simulink model "sampleModel1"  (R2021a)
settings: Solver=VariableStepAuto  StartTime=0.0  StopTime=50  RelTol=1e-3
undefined symbols (not defined in the file): DiscIntNeverNeededParam, magnitude, Newton, Raphson
libraries: simulink x92, pid_lib x10
(part 4 of 5)

== system sampleModel1/cfblk103/cfblk5/cfblk21/cfblk13 ==
  cfblk1 : Inport
  cfblk10 : Sin  TimeSource=Use external signal  SampleTime=0
  cfblk11 : Constant  Value=[-419511582.432887]  SampleTime=1
  cfblk12 : Constant  Value=[-579938406.585944]  SampleTime=1
  cfblk13 : Constant  Value=[41031774.650466]  SampleTime=1
  cfblk14 : Delay
  cfblk15 : Delay
  cfblk16 : Delay
  cfblk3 : simulink/Discrete/Difference  ICPrevInput=0.0  OutMin=[]  OutMax=[]  OutDataTypeStr=Inherit: Inherit via back propagation  OutDataType=fixdt(1, 16)  OutScaling=2^-10  DoSatur=off
  cfblk4 : UnitDelay  SampleTime=-1  HasFrameUpgradeWarning=on
  cfblk5 : Sum  Inputs=+-
  cfblk6 : MinMax  Function=max  Inputs=3
  cfblk7 : ComplexToRealImag
  cfblk8 : simulink/Math Operations/MinMax Running Resettable  Function=min  vinit=0.0
  cfblk9 : MinMax  Function=max  Inputs=2
  cfblk2 : Outport
  wires:
  cfblk4/1 -> cfblk5/1
  cfblk13/1 -> cfblk2/1
  cfblk6/1 -> cfblk7/1
  cfblk11/1 -> cfblk8/1, cfblk6/3
  cfblk9/1 -> cfblk5/2
  cfblk12/1 -> cfblk4/1
  cfblk7/1 -> cfblk8/2
  cfblk7/2 -> cfblk10/1
  cfblk1/1 -> cfblk9/2
  cfblk5/1 -> cfblk3/1
  cfblk3/1 -> cfblk14/1
  cfblk14/1 -> cfblk9/1
  cfblk8/1 -> cfblk15/1
  cfblk15/1 -> cfblk6/1
  cfblk10/1 -> cfblk16/1
  cfblk16/1 -> cfblk6/2

== system sampleModel1/cfblk103/cfblk5/cfblk9/cfblk13 ==
  cfblk1 : Inport
  cfblk3 : Assignment  DiagnosticForDimensions=Warning  IndexOptions=Index vector (dialog)  Indices=1  OutputSizes=1
  cfblk4 : Constant  Value=[323469888.835887]  SampleTime=1
  cfblk5 : Constant  Value=[-52364273.558147]  SampleTime=1
  cfblk2 : Outport
  cfblk6 : Outport  Port=2
  cfblk7 : Outport  Port=3
  wires:
  cfblk5/1 -> cfblk3/1
  cfblk1/1 -> cfblk7/1
  cfblk4/1 -> cfblk6/1, cfblk3/2
  cfblk3/1 -> cfblk2/1

== system sampleModel1/cfblk104/cfblk18/cfblk9/cfblk8 ==
  cfblk1 : Inport
  cfblk13 : Inport  Port=2
  cfblk14 : Inport  Port=3
  cfblk15 : Inport  Port=4
  cfblk10 : Constant  Value=[468184186.952253]  SampleTime=1
  cfblk11 : Constant  Value=[208357491.204136]  SampleTime=1
  cfblk12 : Constant  Value=[-745066327.969250]  SampleTime=1
  cfblk3 : Product  Inputs=*
  cfblk4 : simulink/Math Operations/MinMax Running Resettable  Function=min  vinit=0.0
  cfblk5 : ComplexToMagnitudeAngle
  cfblk6 : DotProduct  InputSameDT=on  OutDataTypeStr=Inherit: Inherit via internal rule
  cfblk7 : PermuteDimensions
  cfblk8 : Constant  Value=[65566875.393897]  SampleTime=1
  cfblk9 : Constant  Value=[546229624.544757]  SampleTime=1
  cfblk2 : Outport
  cfblk16 : Outport  Port=2
  cfblk17 : Outport  Port=3
  wires:
  cfblk10/1 -> cfblk4/1
  cfblk7/1 -> cfblk17/1
  cfblk15/1 -> cfblk2/1
  cfblk5/1 -> cfblk16/1
  cfblk12/1 -> cfblk4/2
  cfblk9/1 -> cfblk6/1
  cfblk1/1 -> cfblk6/2
  cfblk14/1 -> cfblk7/1
  cfblk13/1 -> cfblk3/1
  cfblk3/1 -> cfblk5/1

== system sampleModel1/cfblk104/cfblk19/cfblk17/cfblk12 ==
  cfblk1 : Inport
  cfblk8 : Inport  Port=2
  cfblk9 : Inport  Port=3
  cfblk10 : Inport  Port=4
  cfblk11 : Inport  Port=5
  cfblk12 : Inport  Port=6
  cfblk3 : Sqrt  Operator=rSqrt  AlgorithmType=Newton-Raphson  SaturateOnIntegerOverflow=on
  cfblk4 : PermuteDimensions
  cfblk5 : Assignment  DiagnosticForDimensions=Warning  IndexOptions=Index vector (dialog)  Indices=1  OutputSizes=1
  cfblk6 : Squeeze
  cfblk7 : Constant  Value=[-465349889.808491]  SampleTime=1
  cfblk2 : Outport
  cfblk13 : Outport  Port=2
  wires:
  cfblk5/1 -> cfblk3/1
  cfblk4/1 -> cfblk5/1
  cfblk10/1 -> cfblk2/1
  cfblk8/1 -> cfblk4/1
  cfblk7/1 -> cfblk5/2
  cfblk3/1 -> cfblk13/1
  cfblk12/1 -> cfblk6/1

== system sampleModel1/cfblk104/cfblk19/cfblk17/cfblk13 ==
  cfblk1 : Inport
  cfblk10 : Constant  Value=[70162531.435561]  SampleTime=1
  cfblk11 : Constant  Value=[340915322.911899]  SampleTime=1
  cfblk12 : Constant  Value=[-734252110.443880]  SampleTime=1
  cfblk13 : Constant  Value=[95285484.546552]  SampleTime=1
  cfblk3 : simulink/Discrete/Transfer Fcn Lead or Lag  PoleZ=0.95  ZeroZ=0.75  ICPrevOutput=0.0  ICPrevInput=0.0  DoSatur=off
      settings: SourceProductBaseCode=SL
  cfblk4 : Delay
  cfblk5 : Sqrt  SaturateOnIntegerOverflow=on
  cfblk6 : Sqrt  SaturateOnIntegerOverflow=on
  cfblk7 : Sin  TimeSource=Use external signal  SampleTime=0
  cfblk8 : Sqrt  Operator=rSqrt  AlgorithmType=Newton-Raphson  SaturateOnIntegerOverflow=on
  cfblk9 : Constant  Value=[329230040.299835]  SampleTime=1
  cfblk2 : Outport
  cfblk14 : Outport  Port=2
  wires:
  cfblk11/1 -> cfblk5/1
  cfblk7/1 -> cfblk6/1
  cfblk4/1 -> cfblk2/1
  cfblk9/1 -> cfblk7/1
  cfblk13/1 -> cfblk8/1
  cfblk1/1 -> cfblk14/1
  cfblk3/1 -> cfblk4/1
  cfblk8/1 -> cfblk3/1

== system sampleModel1/cfblk104/cfblk19/cfblk17/cfblk16 ==
  cfblk1 : Inport
  cfblk7 : Inport  Port=2
  Action Port : ActionPort  ActionPortLabel=if(u1 >= 0)
  cfblk3 : ComplexToMagnitudeAngle
  cfblk4 : Reshape
  cfblk5 : ComplexToRealImag
  cfblk6 : Assignment  DiagnosticForDimensions=Warning  IndexOptions=Index vector (dialog)  Indices=1  OutputSizes=1
  cfblk2 : Outport
  wires:
  cfblk4/1 -> cfblk5/1
  cfblk7/1 -> cfblk3/1
  cfblk5/1 -> cfblk6/1
  cfblk5/2 -> cfblk2/1
  cfblk1/1 -> cfblk4/1
  cfblk3/1 -> cfblk6/2

== system sampleModel1/cfblk104/cfblk19/cfblk17/cfblk17 ==
  cfblk1 : Inport
  cfblk9 : Inport  Port=2
  Action Port : ActionPort  ActionPortLabel=else
  cfblk3 : Sum  Inputs=+-
  cfblk4 : Sin  TimeSource=Use external signal  SampleTime=0
  cfblk5 : Squeeze
  cfblk6 : ComplexToRealImag
  cfblk7 : Constant  Value=[-869127634.488702]  SampleTime=1
  cfblk8 : Constant  Value=[403105618.550086]  SampleTime=1
  cfblk2 : Outport
  wires:
  cfblk6/1 -> cfblk2/1
  cfblk8/1 -> cfblk6/1
  cfblk7/1 -> cfblk3/1
  cfblk4/1 -> cfblk5/1
  cfblk1/1 -> cfblk3/2
  cfblk3/1 -> cfblk4/1

== system sampleModel1/cfblk104/cfblk19/cfblk18/cfblk7 ==
  cfblk1 : Inport
  cfblk9 : Inport  Port=2
  cfblk10 : Inport  Port=3
  cfblk11 : Delay
  cfblk3 : DiscreteFir
  cfblk4 : Reshape
  cfblk5 : Sqrt  Operator=rSqrt  AlgorithmType=Newton-Raphson  SaturateOnIntegerOverflow=on
  cfblk6 : Bias  Bias=[-686765959.780988]
  cfblk7 : Constant  Value=[-130705177.150606]  SampleTime=1
  cfblk8 : Constant  Value=[-280180877.090353]  SampleTime=1
  cfblk2 : Outport
  wires:
  cfblk5/1 -> cfblk4/1
  cfblk8/1 -> cfblk2/1
  cfblk3/1 -> cfblk5/1
  cfblk7/1 -> cfblk6/1
  cfblk4/1 -> cfblk11/1
  cfblk11/1 -> cfblk3/1

== system sampleModel1/cfblk104/cfblk21/cfblk11/cfblk11 ==
  cfblk1 : Inport
  cfblk10 : Inport  Port=2
  cfblk11 : Inport  Port=3
  cfblk3 : DiscreteFir
  cfblk4 : UnitDelay  SampleTime=-1  HasFrameUpgradeWarning=on
  cfblk5 : Abs
  cfblk6 : Sin  TimeSource=Use external signal  SampleTime=0
  cfblk7 : Sqrt  SaturateOnIntegerOverflow=on
  cfblk8 : Constant  Value=[815597882.142010]  SampleTime=1
  cfblk9 : Constant  Value=[-760273017.735555]  SampleTime=1
  cfblk2 : Outport
  wires:
  cfblk8/1 -> cfblk6/1
  cfblk11/1 -> cfblk7/1
  cfblk1/1 -> cfblk5/1
  cfblk5/1 -> cfblk3/1
  cfblk3/1 -> cfblk2/1
  cfblk9/1 -> cfblk4/1

== system sampleModel1/cfblk104/cfblk21/cfblk11/cfblk12 ==
  cfblk1 : Inport
  cfblk10 : Constant  Value=[261499476.768893]  SampleTime=1
  cfblk11 : Constant  Value=[-508647636.126222]  SampleTime=1
  cfblk12 : Constant  Value=[-390080084.785966]  SampleTime=1
  cfblk13 : Constant  Value=[-465541815.265822]  SampleTime=1
  cfblk14 : Constant  Value=[-406876444.934026]  SampleTime=1
  cfblk15 : Constant  Value=[938148942.176117]  SampleTime=1
  cfblk16 : Constant  Value=[435762796.775185]  SampleTime=1
  cfblk3 : simulink/Math Operations/MinMax Running Resettable  Function=min  vinit=0.0
  cfblk4 : Sqrt  SaturateOnIntegerOverflow=on
  cfblk5 : Squeeze
  cfblk6 : simulink/Math Operations/Slider Gain  gain=1  low=0  high=2
  cfblk7 : Sqrt  SaturateOnIntegerOverflow=on
  cfblk8 : Product
  cfblk9 : Product  Inputs=*
  cfblk2 : Outport
  cfblk17 : Outport  Port=2
  wires:
  cfblk15/1 -> cfblk6/1
  cfblk8/1 -> cfblk5/1
  cfblk13/1 -> cfblk3/1
  cfblk5/1 -> cfblk7/1
  cfblk3/1 -> cfblk9/1
  cfblk10/1 -> cfblk2/1
  cfblk11/1 -> cfblk8/1
  cfblk12/1 -> cfblk17/1
  cfblk6/1 -> cfblk4/1
  cfblk14/1 -> cfblk3/2
  cfblk4/1 -> cfblk8/2

== system sampleModel1/cfblk104/cfblk21/cfblk12/cfblk12 ==
  cfblk1 : Inport
  Action Port : ActionPort  ActionPortLabel=if(u1 >= 0)
  cfblk11 : Delay
  cfblk3 : UnitDelay  SampleTime=-1  HasFrameUpgradeWarning=on
  cfblk4 : Rounding
  cfblk5 : MinMax  Inputs=3
  cfblk6 : Constant  Value=[890112149.879811]  SampleTime=1
  cfblk7 : Constant  Value=[-865439630.913288]  SampleTime=1
  cfblk8 : Constant  Value=[151495230.431139]  SampleTime=1
  cfblk9 : Constant  Value=[-417103288.097467]  SampleTime=1
  cfblk2 : Outport
  cfblk10 : Outport  Port=2
  wires:
  cfblk5/1 -> cfblk3/1
  cfblk3/1 -> cfblk4/1
  cfblk7/1 -> cfblk2/1
  cfblk9/1 -> cfblk5/1
  cfblk8/1 -> cfblk10/1
  cfblk1/1 -> cfblk5/3
  cfblk4/1 -> cfblk11/1
  cfblk11/1 -> cfblk5/2

== system sampleModel1/cfblk104/cfblk21/cfblk12/cfblk13 ==
  cfblk1 : Inport
  cfblk6 : Inport  Port=2
  cfblk7 : Inport  Port=3
  Action Port : ActionPort  ActionPortLabel=else
  cfblk3 : Product  Inputs=**
  cfblk4 : Constant  Value=[673329880.555540]  SampleTime=1
  cfblk5 : Constant  Value=[46754945.948073]  SampleTime=1
  cfblk2 : Outport
  cfblk8 : Outport  Port=2
  wires:
  cfblk1/1 -> cfblk8/1
  cfblk6/1 -> cfblk3/1
  cfblk4/1 -> cfblk3/2
  cfblk3/1 -> cfblk2/1

== system sampleModel1/cfblk104/cfblk21/cfblk12/cfblk14 ==
  cfblk1 : Inport
  Action Port : ActionPort  ActionPortLabel=if(u1 >= 0)
  cfblk10 : Product  Inputs=*
  cfblk11 : Constant  Value=[442312619.835425]  SampleTime=1
  cfblk12 : Constant  Value=[189723836.537281]  SampleTime=1
  cfblk13 : Constant  Value=[-102397878.841420]  SampleTime=1
  cfblk16 : Delay
  cfblk3 : Product  Inputs=**
  cfblk4 : PermuteDimensions
  cfblk5 : Bias  Bias=[-155918482.521040]
  cfblk6 : Sqrt  SaturateOnIntegerOverflow=on
  cfblk7 : ComplexToRealImag
  cfblk8 : Sqrt  SaturateOnIntegerOverflow=on
  cfblk9 : Product
  cfblk2 : Outport
  cfblk14 : Outport  Port=2
  cfblk15 : Outport  Port=3
  wires:
  cfblk9/1 -> cfblk5/1
  cfblk11/1 -> cfblk4/1
  cfblk13/1 -> cfblk14/1
  cfblk5/1 -> cfblk7/1
  cfblk3/1 -> cfblk2/1
  cfblk12/1 -> cfblk15/1
  cfblk7/1 -> cfblk8/1
  cfblk7/2 -> cfblk10/1
  cfblk4/1 -> cfblk6/1
  cfblk8/1 -> cfblk3/1
  cfblk6/1 -> cfblk3/2
  cfblk1/1 -> cfblk9/2
  cfblk10/1 -> cfblk16/1
  cfblk16/1 -> cfblk9/1

== system sampleModel1/cfblk104/cfblk21/cfblk12/cfblk15 ==
  cfblk1 : Inport
  cfblk13 : Inport  Port=2
  cfblk14 : Inport  Port=3
  cfblk15 : Inport  Port=4
  Action Port : ActionPort  ActionPortLabel=else
  cfblk10 : Constant  Value=[-421838795.697533]  SampleTime=1
  cfblk11 : Constant  Value=[-352587754.567201]  SampleTime=1
  cfblk12 : Constant  Value=[-400732601.566113]  SampleTime=1
  cfblk3 : Squeeze
  cfblk4 : ComplexToRealImag
  cfblk5 : Constant  Value=[-948653583.363454]  SampleTime=1
  cfblk6 : Constant  Value=[-714128839.414161]  SampleTime=1
  cfblk7 : Constant  Value=[251689562.661298]  SampleTime=1
  cfblk8 : Constant  Value=[-55335469.502435]  SampleTime=1
  cfblk9 : Constant  Value=[-770422061.669483]  SampleTime=1
  cfblk2 : Outport
  cfblk16 : Outport  Port=2
  wires:
  cfblk10/1 -> cfblk4/1
  cfblk13/1 -> cfblk16/1
  cfblk4/1 -> cfblk3/1
  cfblk4/2 -> cfblk2/1

== system sampleModel1/cfblk105/cfblk6/cfblk10/cfblk10 ==
  cfblk1 : Inport
  cfblk9 : Inport  Port=2
  cfblk11 : Delay
  cfblk12 : Delay
  cfblk3 : ComplexToMagnitudeAngle
  cfblk4 : Sum  Inputs=-+
  cfblk5 : Reshape
  cfblk6 : Signum
  cfblk7 : Sum  Inputs=--
  cfblk8 : Abs
  cfblk2 : Outport
  cfblk10 : Outport  Port=2
  wires:
  cfblk4/1 -> cfblk6/1
  cfblk1/1 -> cfblk10/1
  cfblk8/1 -> cfblk4/2
  cfblk6/1 -> cfblk5/1
  cfblk3/1 -> cfblk8/1
  cfblk9/1 -> cfblk2/1, cfblk7/2
  cfblk3/2 -> cfblk7/1
  cfblk5/1 -> cfblk11/1
  cfblk11/1 -> cfblk4/1
  cfblk7/1 -> cfblk12/1
  cfblk12/1 -> cfblk3/1

== system sampleModel1/cfblk105/cfblk6/cfblk10/cfblk14 ==
  cfblk1 : Inport
  cfblk12 : Inport  Port=2
  cfblk13 : Inport  Port=3
  cfblk14 : Inport  Port=4
  Action Port : ActionPort  ActionPortLabel=if(u1 >= 0)
  cfblk10 : Constant  Value=[909353169.805887]  SampleTime=1
  cfblk11 : Constant  Value=[-627523588.483763]  SampleTime=1
  cfblk3 : simulink/Discrete/Transfer Fcn First Order  PoleZ=0.95  ICPrevOutput=0.0  DoSatur=off
  cfblk4 : Delay
  cfblk5 : Polyval  Coefs=[ +2.081618890e-019, -1.441693666e-014, +4.719686976e-010, -8.536869453e-006, +1.621573104e-001, -8.087801117e+001 ]
  cfblk6 : Product  Inputs=**
  cfblk7 : Product
  cfblk8 : UnaryMinus
  cfblk9 : Constant  Value=[996327052.148197]  SampleTime=1
  cfblk2 : Outport
  cfblk15 : Outport  Port=2
  cfblk16 : Outport  Port=3
  wires:
  cfblk1/1 -> cfblk3/1
  cfblk3/1 -> cfblk8/1
  cfblk9/1 -> cfblk16/1
  cfblk12/1 -> cfblk5/1
  cfblk7/1 -> cfblk15/1
  cfblk11/1 -> cfblk6/1
  cfblk10/1 -> cfblk7/1
  cfblk14/1 -> cfblk4/1
  cfblk8/1 -> cfblk2/1
  cfblk5/1 -> cfblk7/2
  cfblk13/1 -> cfblk6/2

== system sampleModel1/cfblk105/cfblk6/cfblk10/cfblk15 ==
  cfblk1 : Inport
  cfblk9 : Inport  Port=2
  Action Port : ActionPort  ActionPortLabel=else
  cfblk3 : simulink/Discrete/Transfer Fcn Real Zero  ZeroZ=0.75  ICPrevInput=0.0  DoSatur=off
      settings: SourceProductBaseCode=SL
  cfblk4 : Reshape
  cfblk5 : Reshape
  cfblk6 : Constant  Value=[-408517177.426848]  SampleTime=1
  cfblk7 : Constant  Value=[-412588011.215259]  SampleTime=1
  cfblk8 : Constant  Value=[-308205238.166373]  SampleTime=1
  cfblk2 : Outport
  cfblk10 : Outport  Port=2
  cfblk11 : Outport  Port=3
  wires:
  cfblk3/1 -> cfblk2/1
  cfblk7/1 -> cfblk5/1
  cfblk6/1 -> cfblk3/1
  cfblk8/1 -> cfblk11/1
  cfblk1/1 -> cfblk4/1
  cfblk5/1 -> cfblk10/1

== system sampleModel1/cfblk111/cfblk11/cfblk11/cfblk9 ==
  cfblk1 : Inport
  cfblk9 : Inport  Port=2
  cfblk10 : Delay
  cfblk11 : Delay
  cfblk3 : DotProduct  InputSameDT=on  OutDataTypeStr=Inherit: Inherit via internal rule
  cfblk4 : Sum  Inputs=+
  cfblk5 : Trigonometry
  cfblk6 : Sum
  cfblk7 : Sqrt  Operator=rSqrt  AlgorithmType=Newton-Raphson  SaturateOnIntegerOverflow=on
  cfblk8 : Constant  Value=[680678842.980550]  SampleTime=1
  cfblk2 : Outport
  wires:
  cfblk9/1 -> cfblk3/1
  cfblk3/1 -> cfblk7/1
  cfblk4/1 -> cfblk2/1
  cfblk8/1 -> cfblk4/1
  cfblk1/1 -> cfblk6/2
  cfblk6/1 -> cfblk5/1
  cfblk5/1 -> cfblk10/1
  cfblk10/1 -> cfblk6/1
  cfblk7/1 -> cfblk11/1
  cfblk11/1 -> cfblk3/2

== system sampleModel1/cfblk111/cfblk11/cfblk12/cfblk12 ==
  cfblk1 : Inport
  cfblk11 : Inport  Port=2
  Action Port : ActionPort  ActionPortLabel=if(u1 >= 0)
  cfblk10 : Constant  Value=[246879671.288015]  SampleTime=1
  cfblk3 : Polyval  Coefs=[ +2.081618890e-019, -1.441693666e-014, +4.719686976e-010, -8.536869453e-006, +1.621573104e-001, -8.087801117e+001 ]
  cfblk4 : Sqrt  Operator=rSqrt  AlgorithmType=Newton-Raphson  SaturateOnIntegerOverflow=on
  cfblk5 : Sum  Inputs=--
  cfblk6 : Product
  cfblk7 : Reshape
  cfblk8 : Polyval  Coefs=[ +2.081618890e-019, -1.441693666e-014, +4.719686976e-010, -8.536869453e-006, +1.621573104e-001, -8.087801117e+001 ]
  cfblk9 : Constant  Value=[382037661.110754]  SampleTime=1
  cfblk2 : Outport
  cfblk12 : Outport  Port=2
  cfblk13 : Outport  Port=3
  cfblk14 : Outport  Port=4
  cfblk15 : Outport  Port=5
  wires:
  cfblk7/1 -> cfblk3/1
  cfblk6/1 -> cfblk14/1
  cfblk3/1 -> cfblk12/1
  cfblk11/1 -> cfblk8/1, cfblk5/2
  cfblk8/1 -> cfblk4/1
  cfblk4/1 -> cfblk2/1, cfblk5/1
  cfblk10/1 -> cfblk13/1
  cfblk1/1 -> cfblk6/1, cfblk6/2
  cfblk5/1 -> cfblk15/1
  cfblk9/1 -> cfblk7/1

== system sampleModel1/cfblk111/cfblk11/cfblk12/cfblk13 ==
  cfblk1 : Inport
  cfblk13 : Inport  Port=2
  cfblk14 : Inport  Port=3
  Action Port : ActionPort  ActionPortLabel=else
  cfblk10 : Constant  Value=[360855934.077704]  SampleTime=1
  cfblk11 : Constant  Value=[-216363340.487875]  SampleTime=1
  cfblk12 : Constant  Value=[449040613.713941]  SampleTime=1
  cfblk16 : Delay
  cfblk3 : Product  Inputs=*
  cfblk4 : Reshape
  cfblk5 : Squeeze
  cfblk6 : Sqrt  SaturateOnIntegerOverflow=on
  cfblk7 : Assignment  DiagnosticForDimensions=Warning  IndexOptions=Index vector (dialog)  Indices=1  OutputSizes=1
  cfblk8 : Constant  Value=[339926434.778656]  SampleTime=1
  cfblk9 : Constant  Value=[338991206.712136]  SampleTime=1
  cfblk2 : Outport
  cfblk15 : Outport  Port=2
  wires:
  cfblk8/1 -> cfblk15/1
  cfblk10/1 -> cfblk3/1
  cfblk6/1 -> cfblk2/1
  cfblk5/1 -> cfblk7/1
  cfblk11/1 -> cfblk6/1
  cfblk7/1 -> cfblk4/1
  cfblk1/1 -> cfblk5/1
  cfblk4/1 -> cfblk16/1
  cfblk16/1 -> cfblk7/2

== system sampleModel1/cfblk111/cfblk11/cfblk12/cfblk14 ==
  cfblk1 : Inport
  cfblk9 : Inport  Port=2
  Action Port : ActionPort  ActionPortLabel=if(u1 >= 0)
  cfblk3 : Bias  Bias=[-707875719.304627]
  cfblk4 : Assignment  DiagnosticForDimensions=Warning  IndexOptions=Index vector (dialog)  Indices=1  OutputSizes=1
  cfblk5 : Rounding
  cfblk6 : Trigonometry
  cfblk7 : Constant  Value=[387925857.128569]  SampleTime=1
  cfblk8 : Constant  Value=[-912553202.260724]  SampleTime=1
  cfblk2 : Outport
  cfblk10 : Outport  Port=2
  cfblk11 : Outport  Port=3
  wires:
  cfblk5/1 -> cfblk11/1
  cfblk1/1 -> cfblk4/1
  cfblk7/1 -> cfblk3/1
  cfblk4/1 -> cfblk6/1
  cfblk3/1 -> cfblk5/1
  cfblk6/1 -> cfblk10/1
  cfblk9/1 -> cfblk2/1
  cfblk8/1 -> cfblk4/2

== system sampleModel1/cfblk111/cfblk11/cfblk12/cfblk15 ==
  cfblk1 : Inport
  cfblk8 : Inport  Port=2
  cfblk9 : Inport  Port=3
  cfblk10 : Inport  Port=4
  Action Port : ActionPort  ActionPortLabel=else
  cfblk3 : MinMax
  cfblk4 : Signum
  cfblk5 : Rounding
  cfblk6 : Signum
  cfblk7 : Constant  Value=[527812762.659028]  SampleTime=1
  cfblk2 : Outport
  cfblk11 : Outport  Port=2
  wires:
  cfblk10/1 -> cfblk6/1
  cfblk3/1 -> cfblk11/1
  cfblk8/1 -> cfblk4/1
  cfblk6/1 -> cfblk3/1
  cfblk7/1 -> cfblk5/1
  cfblk4/1 -> cfblk2/1

== system sampleModel1/cfblk111/cfblk11/cfblk6/cfblk8 ==
  cfblk1 : Inport
  cfblk8 : Inport  Port=2
  Action Port : ActionPort  ActionPortLabel=if(u1 >= 0)
  cfblk3 : MinMax  Function=max  Inputs=3
  cfblk4 : simulink/Math Operations/Slider Gain  gain=1  low=0  high=2
  cfblk5 : Gain  Gain=[-580713354.556811]
  cfblk6 : Constant  Value=[-39287024.177822]  SampleTime=1
  cfblk7 : Constant  Value=[-735260719.939917]  SampleTime=1
  cfblk2 : Outport
  wires:
  cfblk6/1 -> cfblk2/1
  cfblk7/1 -> cfblk4/1
  cfblk8/1 -> cfblk5/1
  cfblk5/1 -> cfblk3/1
  cfblk4/1 -> cfblk3/2
  cfblk1/1 -> cfblk3/3

== system sampleModel1/cfblk111/cfblk11/cfblk6/cfblk9 ==
  cfblk1 : Inport
  cfblk9 : Inport  Port=2
  cfblk10 : Inport  Port=3
  cfblk11 : Inport  Port=4
  cfblk12 : Inport  Port=5
  Action Port : ActionPort  ActionPortLabel=else
  cfblk15 : Delay
  cfblk3 : PermuteDimensions
  cfblk4 : Bias  Bias=[939018646.363341]
  cfblk5 : Product  Inputs=*
  cfblk6 : Constant  Value=[-115719020.520580]  SampleTime=1
  cfblk7 : Constant  Value=[-778059505.794407]  SampleTime=1
  cfblk8 : Constant  Value=[-674071793.832320]  SampleTime=1
  cfblk2 : Outport
  cfblk13 : Outport  Port=2
  cfblk14 : Outport  Port=3
  wires:
  cfblk3/1 -> cfblk4/1
  cfblk8/1 -> cfblk14/1
  cfblk4/1 -> cfblk5/1
  cfblk7/1 -> cfblk2/1
  cfblk9/1 -> cfblk13/1
  cfblk5/1 -> cfblk15/1
  cfblk15/1 -> cfblk3/1

== system sampleModel1/cfblk111/cfblk11/cfblk7/cfblk12 ==
  cfblk1 : Inport
  cfblk13 : Inport  Port=2
  cfblk14 : Inport  Port=3
  cfblk15 : Inport  Port=4
  cfblk16 : Inport  Port=5
  cfblk10 : Reshape
  cfblk11 : ComplexToRealImag
  cfblk12 : Constant  Value=[-423829694.747288]  SampleTime=1
  cfblk3 : pid_lib/PID Controller  Controller=PID  Form=Parallel  TimeDomain=Discrete-time  UseExternalTs=off  SampleTime=-1  IntegratorMethod=Forward Euler  FilterMethod=Forward Euler  ControllerParametersSource=internal  P=1  I=1  D=0  UseFilter=on  N=100  TunerSelectOption=Transfer Function Based (PID Tuner App)  InitialConditionSource=internal  InitialConditionForIntegrator=0  InitialConditionForFilter=0  DifferentiatorICPrevScaledInput=0  ExternalReset=none  TrackingMode=off  Kt=1  LimitOutput=off  SatLimitsSource=internal  UpperSaturationLimit=inf  LowerSaturationLimit=-inf  LinearizeAsGain=off  AntiWindupMode=none  Kb=1  POutMin=[]  POutMax=[]  IOutMin=[]  IOutMax=[]  DOutMin=[]  DOutMax=[]  NOutMin=[]  NOutMax=[]  SumOutMin=[]  SumOutMax=[]  SaturationOutMin=[]  SaturationOutMax=[]  PParamMin=[]  PParamMax=[]  IParamMin=[]  IParamMax=[]  DParamMin=[]  DParamMax=[]  NParamMin=[]  NParamMax=[]  KbParamMin=[]  KbParamMax=[]  KtParamMin=[]  KtParamMax=[]  KbOutMin=[]  KbOutMax=[]  KtOutMin=[]  KtOutMax=[]  IntegratorOutMin=[]  IntegratorOutMax=[]  FilterOutMin=[]  FilterOutMax=[]  SumI1OutMin=[]  SumI1OutMax=[]  SumI2OutMin=[]  SumI2OutMax=[]  SumI3OutMin=[]  SumI3OutMax=[]  SumI4OutMin=[]  SumI4OutMax=[]  SumDOutMin=[]  SumDOutMax=[]  DifferentiatorOutMin=[]  DifferentiatorOutMax=[]  FilterDiffOutCoefMin=[]  FilterDiffOutCoefMax=[]  ReciprocalOutMin=[]  ReciprocalOutMax=[]  SumDenOutMin=[]  SumDenOutMax=[]  SumNumOutMin=[]  SumNumOutMax=[]  DivideOutMin=[]  DivideOutMax=[]  UdiffTsProdOutMin=[]  UdiffTsProdOutMax=[]  NTsProdOutMin=[]  NTsProdOutMax=[]  UintegralTsProdOutMin=[]  UintegralTsProdOutMax=[]  UngainTsProdOutMin=[]  UngainTsProdOutMax=[]  IntegratorContinuousStateAttributes=''  IntegratorStateMustResolveToSignalObject=off  IntegratorRTWStateStorageClass=Auto  FilterContinuousStateAttributes=''  FilterStateMustResolveToSignalObject=off  FilterRTWStateStorageClass=Auto  ParallelPVariant=InternalParameters  IdealPVariant=Disabled  IVariant=InternalParameters  DVariant=InternalParameters  IntegratorVariant=Discrete  SatVariant=Disabled  AWVariant=Passthrough  PCopyVariant=Disabled  TRVariant=Disabled  FdbkBlocksVariant=Forward  IdealPFdbkVariant=Disabled  SatFdbkVariant=Disabled  DerivativeFilterVariant=ForwardEulerFilter  NVariant=InternalParameters  NCopyVariant=Disabled  FilterICVariant=InternalICsFilter  IntegratorICVariant=InternalICs  ExternalResetVariant=Disabled  TRSumVariant=Passthrough  SumFdbkVariant=Disabled  SumVariant=Sum_PID  TsampFilterVariant=InternalTs  TsampNgainVariant=Passthrough  TsampIntegralVariant=Passthrough  ExternalSaturationOutDataTypeStr=Inherit: Same as second input
  cfblk4 : DiscreteFir
  cfblk5 : Math  Operator=hypot  SaturateOnIntegerOverflow=on
  cfblk6 : Assignment  DiagnosticForDimensions=Warning  IndexOptions=Index vector (dialog)  Indices=1  OutputSizes=1
  cfblk7 : PermuteDimensions
  cfblk8 : PermuteDimensions
  cfblk9 : Sum  Inputs=-+
  cfblk2 : Outport
  wires:
  cfblk4/1 -> cfblk3/1
  cfblk8/1 -> cfblk7/1
  cfblk11/1 -> cfblk10/1
  cfblk10/1 -> cfblk9/1
  cfblk1/1 -> cfblk2/1
  cfblk9/1 -> cfblk4/1
  cfblk5/1 -> cfblk9/2
  cfblk14/1 -> cfblk6/1
  cfblk11/2 -> cfblk6/2
  cfblk7/1 -> cfblk5/1
  cfblk16/1 -> cfblk11/1
  cfblk13/1 -> cfblk5/2
  cfblk15/1 -> cfblk8/1

== system sampleModel1/cfblk111/cfblk11/cfblk7/cfblk13 ==
  cfblk1 : Inport
  cfblk12 : Inport  Port=2
  cfblk13 : Inport  Port=3
  cfblk10 : Constant  Value=[949658750.222794]  SampleTime=1
  cfblk11 : Constant  Value=[-319797678.233112]  SampleTime=1
  cfblk3 : simulink/Discrete/Transfer Fcn Real Zero  ZeroZ=0.75  ICPrevInput=0.0  DoSatur=off
      settings: SourceProductBaseCode=SL
  cfblk4 : Sqrt  Operator=rSqrt  AlgorithmType=Newton-Raphson  SaturateOnIntegerOverflow=on
  cfblk5 : Abs
  cfblk6 : Math  Operator=log  SaturateOnIntegerOverflow=on
  cfblk7 : Product  Inputs=*
  cfblk8 : Reshape
  cfblk9 : PermuteDimensions
  cfblk2 : Outport
  wires:
  cfblk1/1 -> cfblk4/1
  cfblk12/1 -> cfblk6/1
  cfblk13/1 -> cfblk8/1
  cfblk7/1 -> cfblk3/1
  cfblk5/1 -> cfblk2/1
  cfblk8/1 -> cfblk7/1
  cfblk3/1 -> cfblk5/1
  cfblk11/1 -> cfblk9/1

== system sampleModel1/cfblk112/cfblk11/cfblk13/cfblk15 ==
  cfblk1 : Inport
  cfblk11 : Inport  Port=2
  cfblk12 : Inport  Port=3
  cfblk13 : Inport  Port=4
  cfblk14 : Inport  Port=5
  Action Port : ActionPort  ActionPortLabel=if(u1 >= 0)
  cfblk10 : Constant  Value=[-122266068.845746]  SampleTime=1
  cfblk3 : pid_lib/PID Controller (2DOF)  Controller=PID  Form=Parallel  TimeDomain=Discrete-time  UseExternalTs=off  SampleTime=-1  IntegratorMethod=Forward Euler  FilterMethod=Forward Euler  ControllerParametersSource=internal  P=1  I=1  D=0  UseFilter=on  N=100  b=1  c=1  TunerSelectOption=Transfer Function Based (PID Tuner App)  InitialConditionSource=internal  InitialConditionForIntegrator=0  InitialConditionForFilter=0  DifferentiatorICPrevScaledInput=0  ExternalReset=none  TrackingMode=off  Kt=1  LimitOutput=off  SatLimitsSource=internal  UpperSaturationLimit=inf  LowerSaturationLimit=-inf  LinearizeAsGain=off  AntiWindupMode=none  Kb=1  POutMin=[]  POutMax=[]  IOutMin=[]  IOutMax=[]  DOutMin=[]  DOutMax=[]  NOutMin=[]  NOutMax=[]  bOutMin=[]  bOutMax=[]  cOutMin=[]  cOutMax=[]  SumOutMin=[]  SumOutMax=[]  SaturationOutMin=[]  SaturationOutMax=[]  PParamMin=[]  PParamMax=[]  IParamMin=[]  IParamMax=[]  DParamMin=[]  DParamMax=[]  NParamMin=[]  NParamMax=[]  bParamMin=[]  bParamMax=[]  cParamMin=[]  cParamMax=[]  KbParamMin=[]  KbParamMax=[]  KtParamMin=[]  KtParamMax=[]  KbOutMin=[]  KbOutMax=[]  KtOutMin=[]  KtOutMax=[]  IntegratorOutMin=[]  IntegratorOutMax=[]  FilterOutMin=[]  FilterOutMax=[]  SumI1OutMin=[]  SumI1OutMax=[]  SumI2OutMin=[]  SumI2OutMax=[]  SumI3OutMin=[]  SumI3OutMax=[]  SumI4OutMin=[]  SumI4OutMax=[]  SumDOutMin=[]  SumDOutMax=[]  Sum1OutMin=[]  Sum1OutMax=[]  Sum2OutMin=[]  Sum2OutMax=[]  Sum3OutMin=[]  Sum3OutMax=[]  DifferentiatorOutMin=[]  DifferentiatorOutMax=[]  FilterDiffOutCoefMin=[]  FilterDiffOutCoefMax=[]  ReciprocalOutMin=[]  ReciprocalOutMax=[]  SumDenOutMin=[]  SumDenOutMax=[]  SumNumOutMin=[]  SumNumOutMax=[]  DivideOutMin=[]  DivideOutMax=[]  UdiffTsProdOutMin=[]  UdiffTsProdOutMax=[]  NTsProdOutMin=[]  NTsProdOutMax=[]  UintegralTsProdOutMin=[]  UintegralTsProdOutMax=[]  UngainTsProdOutMin=[]  UngainTsProdOutMax=[]  IntegratorContinuousStateAttributes=''  IntegratorStateMustResolveToSignalObject=off  IntegratorRTWStateStorageClass=Auto  FilterContinuousStateAttributes=''  FilterStateMustResolveToSignalObject=off  FilterRTWStateStorageClass=Auto  ParallelPVariant=InternalParameters  IdealPVariant=Disabled  IVariant=InternalParameters  DVariant=InternalParameters  bVariant=InternalParameters  cVariant=InternalParameters  IntegratorVariant=Discrete  SatVariant=Disabled  AWVariant=Passthrough  PCopyVariant=Disabled  TRVariant=Disabled  FdbkBlocksVariant=Forward  IdealPFdbkVariant=Disabled  SatFdbkVariant=Disabled  DerivativeFilterVariant=ForwardEulerFilter  NVariant=InternalParameters  NCopyVariant=Disabled  FilterICVariant=InternalICsFilter  IntegratorICVariant=InternalICs  ExternalResetVariant=Disabled  TRSumVariant=Passthrough  SumFdbkVariant=Disabled  SumVariant=Sum_PID  TsampFilterVariant=InternalTs  TsampNgainVariant=Passthrough  TsampIntegralVariant=Passthrough  ExternalSaturationOutDataTypeStr=Inherit: Same as second input
      settings: SourceProductBaseCode=SL
  cfblk4 : Delay  DelayLengthSource=Input port
      settings: InputPortMap=u0,p1
  cfblk5 : Squeeze
  cfblk6 : Abs
  cfblk7 : ComplexToMagnitudeAngle
  cfblk8 : Polyval  Coefs=[ +2.081618890e-019, -1.441693666e-014, +4.719686976e-010, -8.536869453e-006, +1.621573104e-001, -8.087801117e+001 ]
  cfblk9 : Constant  Value=[161236866.906013]  SampleTime=1
  cfblk2 : Outport
  cfblk15 : Outport  Port=2
  wires:
  cfblk14/1 -> cfblk3/1
  cfblk12/1 -> cfblk4/1
  cfblk6/1 -> cfblk2/1
  cfblk5/1 -> cfblk3/2
  cfblk11/1 -> cfblk15/1
  cfblk8/1 -> cfblk4/2
  cfblk13/1 -> cfblk6/1
  cfblk9/1 -> cfblk5/1
  cfblk4/1 -> cfblk7/1
  cfblk1/1 -> cfblk8/1

== system sampleModel1/cfblk112/cfblk11/cfblk13/cfblk16 ==
  cfblk1 : Inport
  cfblk8 : Inport  Port=2
  Action Port : ActionPort  ActionPortLabel=else
  cfblk3 : Delay
  cfblk4 : PermuteDimensions
  cfblk5 : Squeeze
  cfblk6 : Constant  Value=[743771143.403290]  SampleTime=1
  cfblk7 : Constant  Value=[-527989586.242749]  SampleTime=1
  cfblk2 : Outport
  cfblk9 : Outport  Port=2
  wires:
  cfblk6/1 -> cfblk4/1
  cfblk1/1 -> cfblk2/1
  cfblk8/1 -> cfblk9/1
  cfblk7/1 -> cfblk3/1
  cfblk4/1 -> cfblk5/1

== system sampleModel1/cfblk112/cfblk11/cfblk14/cfblk14 ==
  cfblk1 : Inport
  Action Port : ActionPort  ActionPortLabel=if(u1 >= 0)
  cfblk3 : Squeeze
  cfblk4 : Bias  Bias=[-497638596.073755]
  cfblk5 : Constant  Value=[875215033.780837]  SampleTime=1
  cfblk6 : Constant  Value=[505821738.043894]  SampleTime=1
  cfblk7 : Constant  Value=[-903146563.627624]  SampleTime=1
  cfblk8 : Constant  Value=[450978110.814705]  SampleTime=1
  cfblk9 : Constant  Value=[265114518.304006]  SampleTime=1
  cfblk2 : Outport
  wires:
  cfblk8/1 -> cfblk4/1
  cfblk4/1 -> cfblk2/1
  cfblk1/1 -> cfblk3/1

== system sampleModel1/cfblk112/cfblk11/cfblk14/cfblk15 ==
  cfblk1 : Inport
  Action Port : ActionPort  ActionPortLabel=else
  cfblk10 : Constant  Value=[818202627.503632]  SampleTime=1
  cfblk11 : Constant  Value=[497271600.581116]  SampleTime=1
  cfblk3 : DiscreteIntegrator  SampleTime=-1  ICPrevOutput=DiscIntNeverNeededParam  ICPrevScaledInput=DiscIntNeverNeededParam
  cfblk4 : Sum  Inputs=|++
  cfblk5 : simulink/Math Operations/Slider Gain  gain=1  low=0  high=2
  cfblk6 : Bias  Bias=[-9164173.785582]
  cfblk7 : Polyval  Coefs=[ +2.081618890e-019, -1.441693666e-014, +4.719686976e-010, -8.536869453e-006, +1.621573104e-001, -8.087801117e+001 ]
  cfblk8 : Signum
  cfblk9 : Constant  Value=[-373032670.560984]  SampleTime=1
  cfblk2 : Outport
  wires:
  cfblk4/1 -> cfblk2/1
  cfblk9/1 -> cfblk6/1
  cfblk1/1 -> cfblk8/1
  cfblk7/1 -> cfblk3/1
  cfblk3/1 -> cfblk4/1
  cfblk6/1 -> cfblk7/1
  cfblk10/1 -> cfblk5/1
  cfblk8/1 -> cfblk4/2

== system sampleModel1/cfblk115/cfblk14/cfblk14/cfblk10 ==
  cfblk1 : Inport
  cfblk12 : Inport  Port=2
  cfblk13 : Inport  Port=3
  cfblk10 : Constant  Value=[352581508.259771]  SampleTime=1
  cfblk11 : Constant  Value=[407353705.186988]  SampleTime=1
  cfblk3 : DiscreteZeroPole  Poles=[0 0.5]  Gain=1  SampleTime=-1
  cfblk4 : Trigonometry
  cfblk5 : Product
  cfblk6 : Constant  Value=[346727033.922065]  SampleTime=1
  cfblk7 : Constant  Value=[-837077149.604303]  SampleTime=1
  cfblk8 : Constant  Value=[-431621581.043910]  SampleTime=1
  cfblk9 : Constant  Value=[-541796869.991993]  SampleTime=1
  cfblk2 : Outport
  cfblk14 : Outport  Port=2
  wires:
  cfblk1/1 -> cfblk5/1
  cfblk13/1 -> cfblk4/1
  cfblk8/1 -> cfblk2/1
  cfblk4/1 -> cfblk14/1
  cfblk3/1 -> cfblk5/2
  cfblk7/1 -> cfblk3/1

== system sampleModel1/cfblk115/cfblk14/cfblk14/cfblk7 ==
  cfblk1 : Inport
  cfblk9 : Inport  Port=2
  cfblk10 : Inport  Port=3
  cfblk11 : Inport  Port=4
  cfblk3 : Delay
  cfblk4 : DiscreteStateSpace  SampleTime=-1
  cfblk5 : Sqrt  SaturateOnIntegerOverflow=on
  cfblk6 : Math  Operator=10^u  SaturateOnIntegerOverflow=on
  cfblk7 : Abs
  cfblk8 : Constant  Value=[421829800.069585]  SampleTime=1
  cfblk2 : Outport
  wires:
  cfblk9/1 -> cfblk7/1
  cfblk11/1 -> cfblk2/1
  cfblk1/1 -> cfblk5/1
  cfblk5/1 -> cfblk6/1
  cfblk4/1 -> cfblk3/1
  cfblk8/1 -> cfblk4/1

== system sampleModel1/cfblk115/cfblk14/cfblk14/cfblk8 ==
  cfblk1 : Inport
  cfblk3 : Sum  Inputs=+-
  cfblk4 : Rounding
  cfblk5 : Product
  cfblk6 : Constant  Value=[931029808.892571]  SampleTime=1
  cfblk7 : Constant  Value=[-506641103.816327]  SampleTime=1
  cfblk8 : Constant  Value=[518610889.480997]  SampleTime=1
  cfblk2 : Outport
  cfblk9 : Outport  Port=2
  wires:
  cfblk8/1 -> cfblk9/1
  cfblk1/1 -> cfblk4/1
  cfblk3/1 -> cfblk2/1
  cfblk6/1 -> cfblk5/1
  cfblk4/1 -> cfblk5/2
  cfblk5/1 -> cfblk3/1
  cfblk7/1 -> cfblk3/2

== system sampleModel1/cfblk115/cfblk14/cfblk14/cfblk9 ==
  cfblk1 : Inport
  cfblk10 : Inport  Port=2
  cfblk11 : Inport  Port=3
  cfblk12 : Inport  Port=4
  cfblk13 : Inport  Port=5
  cfblk3 : Gain  Gain=[407057180.554464]
  cfblk4 : PermuteDimensions
  cfblk5 : Product
  cfblk6 : Product  Inputs=*
  cfblk7 : Math  Operator=hermitian  SaturateOnIntegerOverflow=on
  cfblk8 : Constant  Value=[188349514.589146]  SampleTime=1
  cfblk9 : Constant  Value=[477462067.720349]  SampleTime=1
  cfblk2 : Outport
  wires:
  cfblk8/1 -> cfblk4/1
  cfblk6/1 -> cfblk7/1
  cfblk9/1 -> cfblk5/1
  cfblk1/1 -> cfblk5/2
  cfblk11/1 -> cfblk6/1
  cfblk3/1 -> cfblk2/1
  cfblk10/1 -> cfblk3/1

== system sampleModel1/cfblk115/cfblk14/cfblk9/cfblk11 ==
  cfblk1 : Inport
  cfblk7 : Inport  Port=2
  cfblk3 : Signum
  cfblk4 : Signum
  cfblk5 : Constant  Value=[-157128228.260691]  SampleTime=1
  cfblk6 : Constant  Value=[266854258.418611]  SampleTime=1
  cfblk2 : Outport
  cfblk8 : Outport  Port=2
  wires:
  cfblk5/1 -> cfblk2/1
  cfblk4/1 -> cfblk8/1
  cfblk6/1 -> cfblk4/1
  cfblk1/1 -> cfblk3/1

== system sampleModel1/cfblk73/cfblk18/cfblk11/cfblk12 ==
  cfblk1 : Inport
  cfblk10 : Constant  Value=[966104932.939712]  SampleTime=1
  cfblk3 : DiscreteTransferFcn
  cfblk4 : Polyval  Coefs=[ +2.081618890e-019, -1.441693666e-014, +4.719686976e-010, -8.536869453e-006, +1.621573104e-001, -8.087801117e+001 ]
  cfblk5 : Product  Inputs=**
  cfblk6 : Constant  Value=[840664079.673127]  SampleTime=1
  cfblk7 : Constant  Value=[475716191.033993]  SampleTime=1
  cfblk8 : Constant  Value=[-154328769.982384]  SampleTime=1
  cfblk9 : Constant  Value=[885473968.553869]  SampleTime=1
  cfblk2 : Outport
  cfblk11 : Outport  Port=2
  wires:
  cfblk8/1 -> cfblk5/1
  cfblk7/1 -> cfblk4/1
  cfblk3/1 -> cfblk5/2
  cfblk10/1 -> cfblk2/1
  cfblk1/1 -> cfblk3/1
  cfblk9/1 -> cfblk11/1

== system sampleModel1/cfblk73/cfblk18/cfblk11/cfblk13 ==
  cfblk1 : Inport
  cfblk13 : Inport  Port=2
  cfblk10 : Constant  Value=[759307448.963810]  SampleTime=1
  cfblk11 : Constant  Value=[-478544001.889071]  SampleTime=1
  cfblk12 : Constant  Value=[-954974814.519536]  SampleTime=1
  cfblk3 : Sqrt  Operator=rSqrt  AlgorithmType=Newton-Raphson  SaturateOnIntegerOverflow=on
  cfblk4 : DotProduct  InputSameDT=on  OutDataTypeStr=Inherit: Inherit via internal rule
  cfblk5 : Reshape
  cfblk6 : Squeeze
  cfblk7 : Sin  TimeSource=Use external signal  SampleTime=0
  cfblk8 : Gain  Gain=[168138666.556904]
  cfblk9 : Constant  Value=[-784461969.512514]  SampleTime=1
  cfblk2 : Outport
  cfblk14 : Outport  Port=2
  wires:
  cfblk3/1 -> cfblk4/1
  cfblk7/1 -> cfblk3/1
  cfblk9/1 -> cfblk2/1
  cfblk11/1 -> cfblk6/1
  cfblk10/1 -> cfblk8/1
  cfblk1/1 -> cfblk4/2
  cfblk8/1 -> cfblk5/1
  cfblk6/1 -> cfblk14/1
  cfblk12/1 -> cfblk7/1

== system sampleModel1/cfblk73/cfblk18/cfblk11/cfblk18 ==
  cfblk1 : Inport
  cfblk10 : Inport  Port=2
  Action Port : ActionPort  ActionPortLabel=if(u1 >= 0)
  cfblk11 : Delay
  cfblk3 : simulink/Math Operations/MinMax Running Resettable  Function=min  vinit=0.0
  cfblk4 : Product
  cfblk5 : PermuteDimensions
  cfblk6 : Sum  Inputs=|++
  cfblk7 : Product
  cfblk8 : Constant  Value=[887245249.096776]  SampleTime=1
  cfblk9 : Constant  Value=[915387879.683167]  SampleTime=1
  cfblk2 : Outport
  wires:
  cfblk4/1 -> cfblk6/1
  cfblk8/1 -> cfblk6/2
  cfblk3/1 -> cfblk2/1
  cfblk9/1 -> cfblk3/1
  cfblk5/1 -> cfblk7/1
  cfblk10/1 -> cfblk7/2
  cfblk6/1 -> cfblk3/2, cfblk5/1
  cfblk1/1 -> cfblk4/2
  cfblk7/1 -> cfblk11/1
  cfblk11/1 -> cfblk4/1

== system sampleModel1/cfblk73/cfblk18/cfblk11/cfblk19 ==
  cfblk1 : Inport
  cfblk13 : Inport  Port=2
  cfblk14 : Inport  Port=3
  cfblk15 : Inport  Port=4
  Action Port : ActionPort  ActionPortLabel=else
  cfblk10 : Constant  Value=[288885562.862673]  SampleTime=1
  cfblk11 : Constant  Value=[358033508.186404]  SampleTime=1
  cfblk12 : Constant  Value=[890348226.218803]  SampleTime=1
  cfblk3 : UnitDelay  SampleTime=-1  HasFrameUpgradeWarning=on
  cfblk4 : Signum
  cfblk5 : simulink/Math Operations/Slider Gain  gain=1  low=0  high=2
  cfblk6 : ComplexToRealImag
  cfblk7 : Gain  Gain=[-148542316.257624]
  cfblk8 : Assignment  DiagnosticForDimensions=Warning  IndexOptions=Index vector (dialog)  Indices=1  OutputSizes=1
  cfblk9 : Product  Inputs=*
  cfblk2 : Outport
  wires:
  cfblk5/1 -> cfblk7/1
  cfblk10/1 -> cfblk2/1
  cfblk8/1 -> cfblk5/1
  cfblk13/1 -> cfblk8/1
  cfblk11/1 -> cfblk4/1
  cfblk14/1 -> cfblk6/1
  cfblk3/1 -> cfblk9/1
  cfblk9/1 -> cfblk8/2
  cfblk15/1 -> cfblk3/1

== system sampleModel1/cfblk73/cfblk18/cfblk11/cfblk20 ==
  cfblk1 : Inport
  Action Port : ActionPort  ActionPortLabel=if(u1 >= 0)
  cfblk3 : Rounding
  cfblk4 : Product  Inputs=*
  cfblk5 : Constant  Value=[442093241.159623]  SampleTime=1
  cfblk6 : Constant  Value=[987409248.241704]  SampleTime=1
  cfblk7 : Constant  Value=[-788403453.499544]  SampleTime=1
  cfblk8 : Constant  Value=[-872817258.049789]  SampleTime=1
  cfblk2 : Outport
  cfblk9 : Outport  Port=2
  wires:
  cfblk5/1 -> cfblk3/1
  cfblk6/1 -> cfblk9/1
  cfblk8/1 -> cfblk4/1
  cfblk1/1 -> cfblk2/1

== system sampleModel1/cfblk73/cfblk18/cfblk11/cfblk21 ==
  cfblk1 : Inport
  cfblk8 : Inport  Port=2
  Action Port : ActionPort  ActionPortLabel=else
  cfblk3 : MinMax  Function=max  Inputs=3
  cfblk4 : Constant  Value=[40104934.780774]  SampleTime=1
  cfblk5 : Constant  Value=[-700005492.336634]  SampleTime=1
  cfblk6 : Constant  Value=[-475709364.544385]  SampleTime=1
  cfblk7 : Constant  Value=[509866534.462358]  SampleTime=1
  cfblk2 : Outport
  wires:
  cfblk6/1 -> cfblk2/1
  cfblk7/1 -> cfblk3/1
  cfblk5/1 -> cfblk3/2
  cfblk4/1 -> cfblk3/3

== system sampleModel1/cfblk73/cfblk18/cfblk12/cfblk8 ==
  cfblk1 : Inport
  cfblk9 : Inport  Port=2
  cfblk10 : Inport  Port=3
  cfblk11 : Inport  Port=4
  Action Port : ActionPort  ActionPortLabel=if(u1 >= 0)
  cfblk3 : DotProduct  InputSameDT=on  OutDataTypeStr=Inherit: Inherit via internal rule
  cfblk4 : Constant  Value=[332832434.638936]  SampleTime=1
  cfblk5 : Constant  Value=[251919570.343167]  SampleTime=1
  cfblk6 : Constant  Value=[459503710.634442]  SampleTime=1
  cfblk7 : Constant  Value=[964606445.767213]  SampleTime=1
  cfblk8 : Constant  Value=[162892975.750796]  SampleTime=1
  cfblk2 : Outport
  cfblk12 : Outport  Port=2
  cfblk13 : Outport  Port=3
  wires:
  cfblk1/1 -> cfblk12/1
  cfblk10/1 -> cfblk2/1
  cfblk9/1 -> cfblk3/1
  cfblk7/1 -> cfblk3/2
  cfblk3/1 -> cfblk13/1

== system sampleModel1/cfblk73/cfblk18/cfblk12/cfblk9 ==
  cfblk1 : Inport
  Action Port : ActionPort  ActionPortLabel=else
  cfblk10 : Sum  Inputs=|++
  cfblk11 : Product  Inputs=**
  cfblk12 : Constant  Value=[-588048968.935513]  SampleTime=1
  cfblk13 : Constant  Value=[-835857585.804548]  SampleTime=1
  cfblk14 : Delay
  cfblk3 : DiscreteIntegrator  SampleTime=-1  ICPrevOutput=DiscIntNeverNeededParam  ICPrevScaledInput=DiscIntNeverNeededParam
  cfblk4 : DiscreteStateSpace  SampleTime=-1
  cfblk5 : Product  Inputs=*
  cfblk6 : PermuteDimensions
  cfblk7 : Bias  Bias=[129959141.476402]
  cfblk8 : Polyval  Coefs=[ +2.081618890e-019, -1.441693666e-014, +4.719686976e-010, -8.536869453e-006, +1.621573104e-001, -8.087801117e+001 ]
  cfblk9 : Sum  Inputs=+-
  cfblk2 : Outport
  wires:
  cfblk4/1 -> cfblk3/1
  cfblk9/1 -> cfblk8/1
  cfblk13/1 -> cfblk2/1
  cfblk8/1 -> cfblk10/1
  cfblk11/1 -> cfblk4/1
  cfblk12/1 -> cfblk11/1
  cfblk7/1 -> cfblk11/2
  cfblk1/1 -> cfblk7/1, cfblk10/2
  cfblk3/1 -> cfblk6/1
  cfblk10/1 -> cfblk5/1
  cfblk6/1 -> cfblk9/2
  cfblk5/1 -> cfblk14/1
  cfblk14/1 -> cfblk9/1

== system sampleModel1/cfblk89/cfblk11/cfblk13/cfblk9 ==
  cfblk1 : Inport
  cfblk10 : Delay
  cfblk3 : ComplexToRealImag
  cfblk4 : Product  Inputs=**
  cfblk5 : Product  Inputs=**
  cfblk6 : Sum  Inputs=+
  cfblk7 : Sum  Inputs=+
  cfblk8 : ComplexToMagnitudeAngle
  cfblk9 : Delay
  cfblk2 : Outport
  wires:
  cfblk1/1 -> cfblk4/1
  cfblk5/1 -> cfblk6/1
  cfblk4/1 -> cfblk8/1
  cfblk3/1 -> cfblk5/1
  cfblk8/1 -> cfblk7/1
  cfblk7/1 -> cfblk2/1
  cfblk3/2 -> cfblk5/2
  cfblk8/2 -> cfblk9/1
  cfblk9/1 -> cfblk4/2
  cfblk6/1 -> cfblk10/1
  cfblk10/1 -> cfblk3/1

== system sampleModel1/cfblk89/cfblk11/cfblk14/cfblk5 ==
  cfblk1 : Inport
  cfblk11 : Inport  Port=2
  cfblk10 : Constant  Value=[-169813226.773907]  SampleTime=1
  cfblk3 : UnaryMinus
  cfblk4 : Product  Inputs=*
  cfblk5 : Signum
  cfblk6 : Sum  Inputs=-+
  cfblk7 : Squeeze
  cfblk8 : Constant  Value=[50090329.525218]  SampleTime=1
  cfblk9 : Constant  Value=[92898879.806137]  SampleTime=1
  cfblk2 : Outport
  cfblk12 : Outport  Port=2
  wires:
  cfblk1/1 -> cfblk3/1
  cfblk8/1 -> cfblk12/1
  cfblk4/1 -> cfblk7/1
  cfblk10/1 -> cfblk6/1
  cfblk7/1 -> cfblk5/1
  cfblk9/1 -> cfblk2/1
  cfblk3/1 -> cfblk4/1
  cfblk11/1 -> cfblk6/2

== system sampleModel1/cfblk91/cfblk16/cfblk16/cfblk12 ==
  cfblk1 : Inport
  cfblk16 : Inport  Port=2
  Action Port : ActionPort  ActionPortLabel=if(u1 >= 0)
  cfblk10 : Trigonometry
  cfblk11 : Constant  Value=[89811796.489343]  SampleTime=1
  cfblk12 : Constant  Value=[787265391.867203]  SampleTime=1
  cfblk13 : Constant  Value=[-392677240.565968]  SampleTime=1
  cfblk14 : Constant  Value=[-609046472.732403]  SampleTime=1
  cfblk15 : Constant  Value=[443506546.998594]  SampleTime=1
  cfblk3 : DiscreteFir
  cfblk4 : MinMax  Inputs=2
  cfblk5 : ComplexToMagnitudeAngle
  cfblk6 : Math  Operator=rem  SaturateOnIntegerOverflow=on
  cfblk7 : Bias  Bias=[589364314.667610]
  cfblk8 : Sum  Inputs=|++
  cfblk9 : Assignment  DiagnosticForDimensions=Warning  IndexOptions=Index vector (dialog)  Indices=1  OutputSizes=1
  cfblk2 : Outport
  cfblk17 : Outport  Port=2
  wires:
  cfblk1/1 -> cfblk7/1
  cfblk14/1 -> cfblk17/1
  cfblk10/1 -> cfblk4/1
  cfblk12/1 -> cfblk10/1
  cfblk7/1 -> cfblk8/1
  cfblk11/1 -> cfblk5/1
  cfblk13/1 -> cfblk3/1
  cfblk9/1 -> cfblk6/1
  cfblk3/1 -> cfblk4/2
  cfblk5/1 -> cfblk6/2
  cfblk15/1 -> cfblk9/1
  cfblk4/1 -> cfblk9/2
  cfblk8/1 -> cfblk2/1
  cfblk16/1 -> cfblk8/2

== system sampleModel1/cfblk91/cfblk16/cfblk16/cfblk13 ==
  cfblk1 : Inport
  cfblk12 : Inport  Port=2
  cfblk13 : Inport  Port=3
  Action Port : ActionPort  ActionPortLabel=else
  cfblk10 : Constant  Value=[621900064.476530]  SampleTime=1
  cfblk11 : Constant  Value=[513498420.131024]  SampleTime=1
  cfblk3 : simulink/Discrete/Transfer Fcn Lead or Lag  PoleZ=0.95  ZeroZ=0.75  ICPrevOutput=0.0  ICPrevInput=0.0  DoSatur=off
      settings: SourceProductBaseCode=SL
  cfblk4 : Sum  Inputs=+-
  cfblk5 : Sqrt  Operator=rSqrt  AlgorithmType=Newton-Raphson  SaturateOnIntegerOverflow=on
  cfblk6 : Constant  Value=[867003217.014210]  SampleTime=1
  cfblk7 : Constant  Value=[-586447084.129790]  SampleTime=1
  cfblk8 : Constant  Value=[-855896897.558700]  SampleTime=1
  cfblk9 : Constant  Value=[333863066.414997]  SampleTime=1
  cfblk2 : Outport
  cfblk14 : Outport  Port=2
  cfblk15 : Outport  Port=3
  cfblk16 : Outport  Port=4
  cfblk17 : Outport  Port=5
  wires:
  cfblk13/1 -> cfblk17/1
  cfblk6/1 -> cfblk16/1
  cfblk5/1 -> cfblk4/1
  cfblk11/1 -> cfblk14/1
  cfblk8/1 -> cfblk15/1
  cfblk1/1 -> cfblk4/2
  cfblk7/1 -> cfblk5/1
  cfblk12/1 -> cfblk2/1
  cfblk10/1 -> cfblk3/1

== system sampleModel1/cfblk91/cfblk16/cfblk16/cfblk14 ==
  cfblk1 : Inport
  cfblk9 : Inport  Port=2
  Action Port : ActionPort  ActionPortLabel=if(u1 >= 0)
  cfblk3 : Squeeze
  cfblk4 : MinMax  Function=max  Inputs=2
  cfblk5 : Polyval  Coefs=[ +2.081618890e-019, -1.441693666e-014, +4.719686976e-010, -8.536869453e-006, +1.621573104e-001, -8.087801117e+001 ]
  cfblk6 : Sum  Inputs=+-
  cfblk7 : Constant  Value=[-347915658.154417]  SampleTime=1
  cfblk8 : Constant  Value=[427591166.466269]  SampleTime=1
  cfblk2 : Outport
  cfblk10 : Outport  Port=2
  wires:
  cfblk1/1 -> cfblk6/1
  cfblk5/1 -> cfblk6/2
  cfblk3/1 -> cfblk4/1
  cfblk6/1 -> cfblk10/1
  cfblk7/1 -> cfblk2/1
  cfblk9/1 -> cfblk4/2
  cfblk4/1 -> cfblk5/1
  cfblk8/1 -> cfblk3/1

== system sampleModel1/cfblk91/cfblk16/cfblk16/cfblk15 ==
  cfblk1 : Inport
  cfblk12 : Inport  Port=2
  cfblk13 : Inport  Port=3
  Action Port : ActionPort  ActionPortLabel=else
  cfblk10 : Product  Inputs=*
  cfblk11 : Constant  Value=[775478431.065432]  SampleTime=1
  cfblk15 : Delay
  cfblk3 : simulink/Discrete/Difference  ICPrevInput=0.0  OutMin=[]  OutMax=[]  OutDataTypeStr=Inherit: Inherit via back propagation  OutDataType=fixdt(1, 16)  OutScaling=2^-10  DoSatur=off
  cfblk4 : DiscreteTransferFcn
  cfblk5 : Reshape
  cfblk6 : Sum  Inputs=+-
  cfblk7 : Product
  cfblk8 : simulink/Math Operations/MinMax Running Resettable  Function=min  vinit=0.0
  cfblk9 : Polyval  Coefs=[ +2.081618890e-019, -1.441693666e-014, +4.719686976e-010, -8.536869453e-006, +1.621573104e-001, -8.087801117e+001 ]
  cfblk2 : Outport
  cfblk14 : Outport  Port=2
  wires:
  cfblk12/1 -> cfblk6/1
  cfblk9/1 -> cfblk5/1
  cfblk11/1 -> cfblk10/1
  cfblk3/1 -> cfblk14/1, cfblk8/2
  cfblk13/1 -> cfblk3/1
  cfblk6/1 -> cfblk7/1
  cfblk10/1 -> cfblk7/2
  cfblk4/1 -> cfblk6/2
  cfblk7/1 -> cfblk9/1
  cfblk1/1 -> cfblk8/1
  cfblk8/1 -> cfblk2/1
  cfblk5/1 -> cfblk15/1
  cfblk15/1 -> cfblk4/1

== system sampleModel1/cfblk91/cfblk18/cfblk14/cfblk10 ==
  cfblk1 : Inport
  Action Port : ActionPort  ActionPortLabel=if(u1 >= 0)
  cfblk3 : DiscreteIntegrator  SampleTime=-1  ICPrevOutput=DiscIntNeverNeededParam  ICPrevScaledInput=DiscIntNeverNeededParam
  cfblk4 : Gain  Gain=[812886533.020004]
  cfblk5 : UnaryMinus
  cfblk6 : Constant  Value=[-214630848.051777]  SampleTime=1
  cfblk7 : Constant  Value=[342873593.144920]  SampleTime=1
  cfblk8 : Constant  Value=[942999276.622527]  SampleTime=1
  cfblk2 : Outport
  wires:
  cfblk6/1 -> cfblk3/1
  cfblk7/1 -> cfblk5/1
  cfblk5/1 -> cfblk4/1
  cfblk4/1 -> cfblk2/1

== system sampleModel1/cfblk91/cfblk18/cfblk14/cfblk11 ==
  cfblk1 : Inport
  Action Port : ActionPort  ActionPortLabel=else
  cfblk3 : DiscreteZeroPole  Poles=[0 0.5]  Gain=1  SampleTime=-1
  cfblk4 : Math  Operator=square  SaturateOnIntegerOverflow=on
  cfblk5 : Trigonometry
  cfblk6 : Constant  Value=[-453566584.000073]  SampleTime=1
  cfblk2 : Outport
  cfblk7 : Outport  Port=2
  cfblk8 : Outport  Port=3
  wires:
  cfblk3/1 -> cfblk4/1
  cfblk4/1 -> cfblk2/1, cfblk7/1
  cfblk5/1 -> cfblk3/1
  cfblk6/1 -> cfblk5/1
  cfblk1/1 -> cfblk8/1

== system sampleModel1/cfblk91/cfblk18/cfblk15/cfblk10 ==
  cfblk1 : Inport
  cfblk11 : Inport  Port=2
  cfblk12 : Inport  Port=3
  Action Port : ActionPort  ActionPortLabel=else
  cfblk10 : Constant  Value=[141982150.924811]  SampleTime=1
  cfblk15 : Delay
  cfblk3 : DiscreteFir
  cfblk4 : Squeeze
  cfblk5 : ComplexToRealImag
  cfblk6 : simulink/Math Operations/MinMax Running Resettable  Function=min  vinit=0.0
  cfblk7 : MinMax  Function=max  Inputs=3
  cfblk8 : Constant  Value=[-584793931.240039]  SampleTime=1
  cfblk9 : Constant  Value=[-732378029.287748]  SampleTime=1
  cfblk2 : Outport
  cfblk13 : Outport  Port=2
  cfblk14 : Outport  Port=3
  wires:
  cfblk8/1 -> cfblk14/1
  cfblk1/1 -> cfblk2/1
  cfblk6/1 -> cfblk13/1
  cfblk11/1 -> cfblk5/1
  cfblk9/1 -> cfblk6/1
  cfblk12/1 -> cfblk7/1
  cfblk5/1 -> cfblk4/1
  cfblk3/1 -> cfblk7/2
  cfblk5/2 -> cfblk7/3
  cfblk4/1 -> cfblk6/2
  cfblk7/1 -> cfblk15/1
  cfblk15/1 -> cfblk3/1

== system sampleModel1/cfblk91/cfblk18/cfblk15/cfblk11 ==
  cfblk1 : Inport
  cfblk10 : Inport  Port=2
  cfblk11 : Inport  Port=3
  cfblk12 : Inport  Port=4
  cfblk13 : Inport  Port=5
  Action Port : ActionPort  ActionPortLabel=if(u1 >= 0)
  cfblk3 : Sum  Inputs=+
  cfblk4 : ComplexToRealImag
  cfblk5 : simulink/Math Operations/MinMax Running Resettable  Function=min  vinit=0.0
  cfblk6 : Sin  TimeSource=Use external signal  SampleTime=0
  cfblk7 : Constant  Value=[-921631026.704834]  SampleTime=1
  cfblk8 : Constant  Value=[527346647.327522]  SampleTime=1
  cfblk9 : Constant  Value=[-632314111.068451]  SampleTime=1
  cfblk2 : Outport
  cfblk14 : Outport  Port=2
  cfblk15 : Outport  Port=3
  wires:
  cfblk13/1 -> cfblk5/1
  cfblk12/1 -> cfblk14/1
  cfblk5/1 -> cfblk6/1
  cfblk7/1 -> cfblk15/1
  cfblk6/1 -> cfblk2/1
  cfblk8/1 -> cfblk5/2
  cfblk11/1 -> cfblk4/1
  cfblk9/1 -> cfblk3/1
